simulink model "Series_RLC_differen"  (R2023a)
settings: Solver=VariableStepAuto  StartTime=0.0  StopTime=10.0  RelTol=1e-3
libraries: spspowerguiLib x1
settings Model: Creator=Ganesh Fashion  LastModifiedBy=Ganesh Fashion

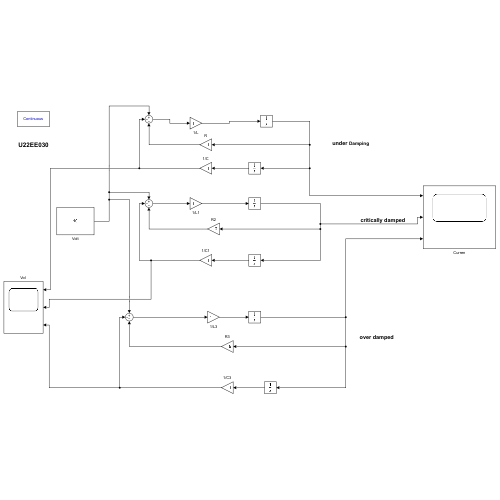
[thumbnail: Simulink's stored preview of the top-level diagram]
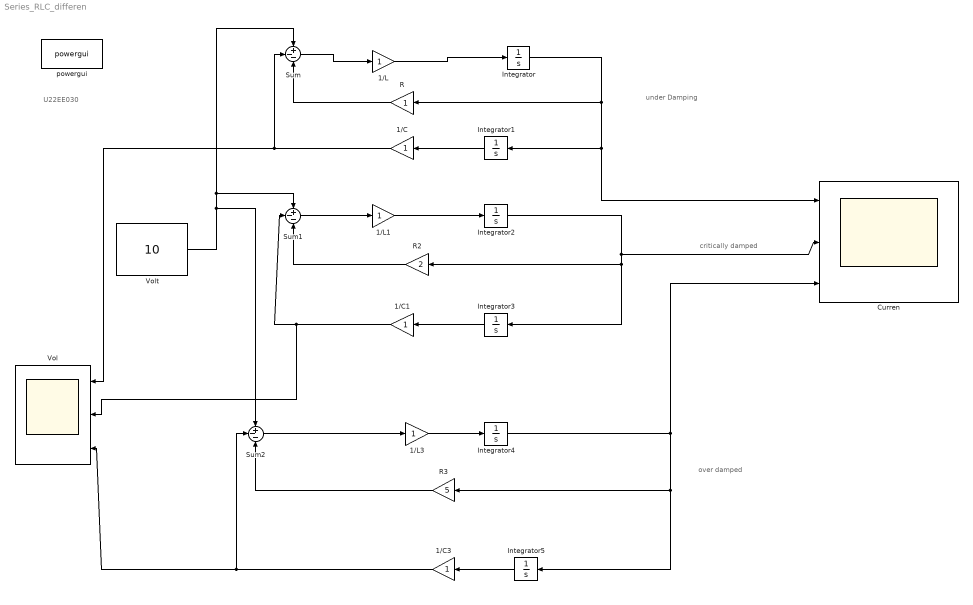
== system Series_RLC_differen ==
  note: U22EE030
  note: over damped
  note: critically damped
  note: under Damping
  1/C : Gain
  1/C1 : Gain
  1/C3 : Gain
  1/L : Gain
  1/L1 : Gain
  1/L3 : Gain
  Curren : Scope  NumInputPorts=3
  Integrator{,1..5} (6 alike) : Integrator
  R : Gain
  R2 : Gain  Gain=2
  R3 : Gain  Gain=5
  Sum : Sum  Inputs=+--
  Sum1 : Sum  Inputs=+--
  Sum2 : Sum  Inputs=+--
  "Vol " : Scope  NumInputPorts=3
  Volt : Constant  Value=10
  powergui : spspowerguiLib/powergui  Priority=1  SimulationMode=Continuous  SampleTime=50e-6  frequency=60  Iterations=50  frequencyindice=60  Pbase=100e6  ErrMax=1e-4  UnitsV=kV  UnitsW=MW  buscounter=0  FunctionMessages=off  echomessages=off  EnableUseOfTLC=off  CurrentSourceSwitches=off  DisableSnubberDevices=off  DisableRonSwitches=off  DisableVfSwitches=off  DisplayEquations=off  AutomaticDiscreteSolvers=off  SolverType=Tustin/Backward Euler (TBE)  Interpol=off  ExternalGateDelay=off  methode=off  Ts=100  x0status=blocks  SPID=on  SwTol=0  HookPort=off  NonlinearTolerance=1e-4  nMaxIteration=100  ContinueOnMaxIteration=off  RestoreLinks=warning  ResistiveCurrentMeasurement=off  Frange=[0:2:500]  Ylog=off  Xlog=on  ShowGrid=off  save=off  variable=ZData  structure=0  ZoomFFT=off  StartTime=0.0  cycles=1  DisplayStyle=1  fundamental=60  FreqAxis=off  MaxFrequency=1000  frequencyindicesteady=1  RmsSteady=1  display=off
  wires:
  1/L/1 -> Integrator/1
  Integrator/1 -> Integrator1/1, Curren/1, R/1
  Sum/1 -> 1/L/1
  R/1 -> Sum/3
  Integrator1/1 -> 1/C/1
  1/C/1 -> "Vol "/1, Sum/2
  Sum1/1 -> 1/L1/1
  1/L1/1 -> Integrator2/1
  R2/1 -> Sum1/3
  1/C1/1 -> "Vol "/2, Sum1/2
  Integrator2/1 -> Curren/2, Integrator3/1, R2/1
  Integrator3/1 -> 1/C1/1
  Sum2/1 -> 1/L3/1
  1/L3/1 -> Integrator4/1
  R3/1 -> Sum2/3
  1/C3/1 -> Sum2/2, "Vol "/3
  Integrator5/1 -> 1/C3/1
  Integrator4/1 -> Curren/3, Integrator5/1, R3/1
  Volt/1 -> Sum2/1, Sum/1, Sum1/1
